simulink model "dynamics_with_control"  (R2023b)
settings: Solver=ode45  StartTime=0.0  StopTime=StopTime  FixedStep=.1  RelTol=1e-5
PreLoadFcn:
  | gravity = true;
  | e_a = 504;
  | e_b = 496;
  | k = 10;
  | b = 10;
  | ktr = 10;
  | btr = 10;
  | ks = 0.1;
  | bs = 10;
  | d0 = 125;
  | l0 = 615.3882;
  | p0 = 100;
  | ls0 = 707.1068;
  | w = -0.007;
  | kp_M = 0.1;
  | ki_M = 0.0023;
  | mu = 398600000000000;
  | mp = 1500;
  | mp_inv = 0.00066667;
  | mtr = 1.6667;
  | mtr_inv = 0.6;
  | NRao0 = [499.999999999579;-4.21217266566732e-10;6878000];
  | NRbo0 = [-500.000000000421;-4.21094801886817e-10;6878000];
  | NRfo0 = [-4.21186650396753e-10;-4.21186650396753e-10;6878500];
  | NRgo0 = [-4.21125418056796e-10;-4.21125418056796e-10;6877500];
  | NRdo0 = [-4.21171342311764e-10;-125.000000000421;6878000];
  | NReo0 = [-4.21140726141785e-10;124.999999999579;6878000];
  | NVao0 = [7612.67977015526;-9.32070078155593e-13;-3.49999999999953];
  | NVbo0 = [7612.67977015526;-9.32498704535295e-13;3.50000000000047];
  | NVfo0 = [7616.17977015526;-9.32713017725146e-13;4.66356508862573e-13];
  | NVgo0 = [7609.17977015526;-9.31855764965743e-13;4.65927882482871e-13];
  | NVdo0 = [7612.67977015526;-9.32284391345444e-13;4.66142195672722e-13];
  | NVeo0 = [7612.67977015526;-9.32284391345444e-13;4.66142195672722e-13];
PostLoadFcn:
  | StopTime = 3000;
values from neighbouring files (symbols this model uses):
  truss_length = 250    [main.m]
libraries: matrix_library x16, vrlib x14
(part 1 of 2)
settings Model: Creator=cyrus  LastModifiedBy=cyrus

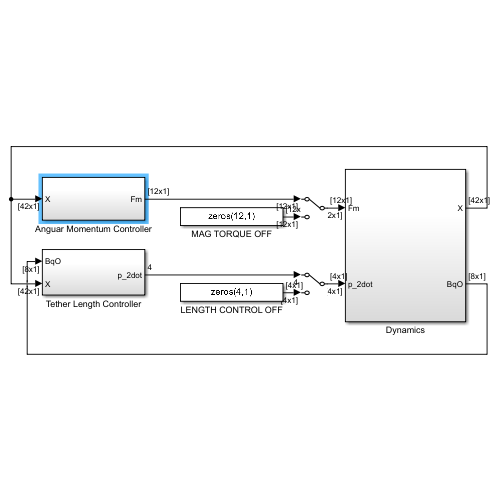
[thumbnail: Simulink's stored preview of the top-level diagram]
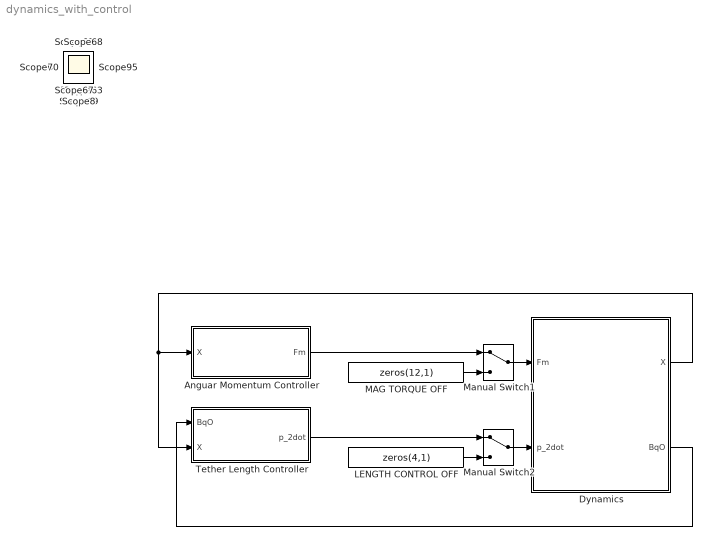
== system dynamics_with_control ==
  Anguar Momentum Controller : Subsystem
  Dynamics : Subsystem
  LENGTH CONTROL OFF : Constant  Value=zeros(4,1)  VectorParams1D=off
  MAG TORQUE OFF : Constant  Value=zeros(12,1)  VectorParams1D=off
  Manual Switch1 : ManualSwitch
  Manual Switch2 : ManualSwitch
  Tether Length Controller : Subsystem
  Scope{,1..36,38,40..70} (69 alike) : Scope
  wires:
  Dynamics/1(X) -> Anguar Momentum Controller/1(X), Tether Length Controller/2(X)
  Manual Switch1/1 -> Dynamics/1(Fm)
  Anguar Momentum Controller/1(Fm) -> Manual Switch1/1
  MAG TORQUE OFF/1 -> Manual Switch1/2
  Manual Switch2/1 -> Dynamics/2(p_2dot)
  LENGTH CONTROL OFF/1 -> Manual Switch2/2
  Tether Length Controller/1(p_2dot) -> Manual Switch2/1
  Dynamics/2(BqO) -> Tether Length Controller/1(BqO)

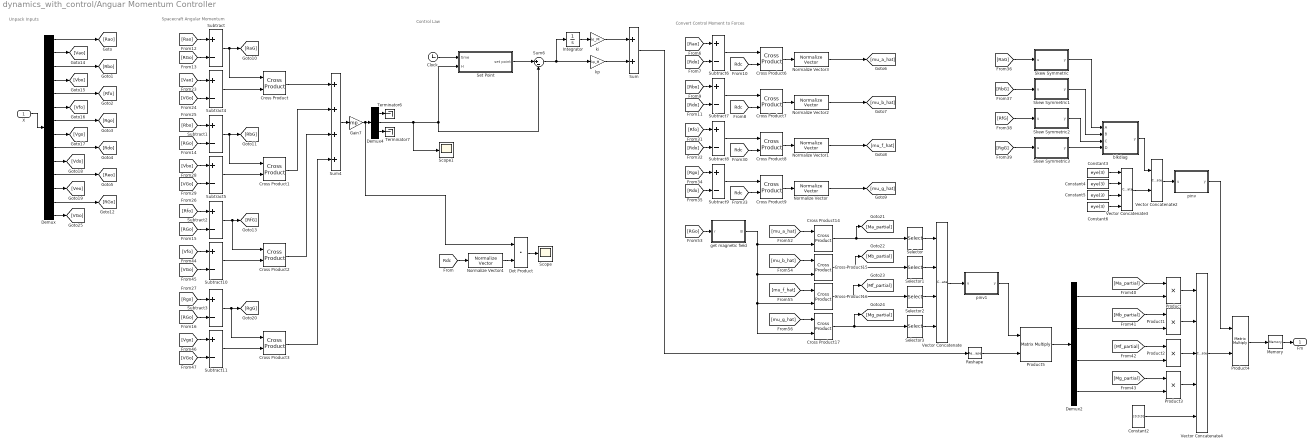
== system dynamics_with_control/Anguar Momentum Controller ==
  note: Convert Control Moment to Forces
  note: Control Law
  note: Spacecraft Angular Momentum
  note: Unpack Inputs
  X : Inport
  Clock : Clock
  Constant2 : Constant  Value=[0;0;0]  VectorParams1D=off
  Constant{3..6} (4 alike) : Constant  Value=eye(3)  VectorParams1D=off
  Cross Product{,1..3,6..9,14..17} (12 alike) : matrix_library/Cross Product
  Demux : Demux  Outputs=14
  Demux2 : Demux
  Demux4 : Demux  Outputs=3
  Dot Product : DotProduct  OutDataTypeStr=Inherit: Inherit via internal rule
  Gain7 : Gain  Gain=mp
  Integrator : Integrator
  Memory : Memory
  Normalize Vector{,1..4} (5 alike) : vrlib/Utilities/Normalize Vector  maxzero=0
  Product{,1..3} (4 alike) : Product
  Product4 : Product  Multiplication=Matrix(*)
  Product5 : Product  Multiplication=Matrix(*)
  Reshape : Reshape  OutputDimensionality=Customize
  Scope : Scope
  Scope1 : Scope
  Selector{,1..3} (4 alike) : Selector  InputPortWidth=3  IndexOptions=Index vector (dialog)  Indices=2  OutputSizes=1
  Set Point : Subsystem
  Skew Symmetric : MATLAB Function  TreatAsAtomicUnit=on
  Skew Symmetric1 : MATLAB Function  TreatAsAtomicUnit=on
  Skew Symmetric2 : MATLAB Function  TreatAsAtomicUnit=on
  Skew Symmetric3 : MATLAB Function  TreatAsAtomicUnit=on
  Subtract{,1..11} (12 alike) : Sum  Inputs=+-
  Sum : Sum
  Sum4 : Sum  Inputs=++++
  Sum6 : Sum  Inputs=|+-
  Terminator6 : Terminator
  Terminator7 : Terminator
  Vector Concatenate : Concatenate  NumInputs=4  Mode=Multidimensional array  ConcatenateDimension=2
  Vector Concatenate2 : Concatenate  Mode=Multidimensional array
  Vector Concatenate3 : Concatenate  NumInputs=4  Mode=Multidimensional array  ConcatenateDimension=2
  Vector Concatenate4 : Concatenate  NumInputs=5
  blkdiag : MATLAB Function  TreatAsAtomicUnit=on
  get magnetic field : MATLAB Function  TreatAsAtomicUnit=on
  ki : Gain  Gain=ki_M
  kp : Gain  Gain=kp_M
  pinv : MATLAB Function  TreatAsAtomicUnit=on
  pinv1 : MATLAB Function  TreatAsAtomicUnit=on
  Fm : Outport
  wires:
  X/1 -> Demux/1
  Sum6/1 -> Integrator/1, kp/1
  Integrator/1 -> ki/1
  ki/1 -> Sum/1
  [RGo] -> Subtract1/2
  Demux/4 -> [Vbo]
  Demux/9 -> [Rdo]
  Demux/2 -> [Vao]
  Subtract3/1 -> Cross Product3/1, [RgG]
  Demux/8 -> [Vgo]
  Demux/10 -> [Vdo]
  Demux/12 -> [Veo]
  Demux/5 -> [Rfo]
  Subtract/1 -> [RaG], Cross Product/1
  Demux/3 -> [Rbo]
  [RGo] -> Subtract3/2
  Demux/7 -> [Rgo]
  Demux/6 -> [Vfo]
  [Rfo] -> Subtract2/1
  Demux/1 -> [Rao]
  [Rbo] -> Subtract1/1
  [RGo] -> Subtract/2
  [Rao] -> Subtract/1
  Subtract1/1 -> Cross Product1/1, [RbG]
  Subtract2/1 -> Cross Product2/1, [RfG]
  Demux/11 -> [Reo]
  [Rgo] -> Subtract3/1
  [RGo] -> Subtract2/2
  [Rdo] -> Subtract6/2
  [Rao] -> Subtract6/1
  Subtract6/1 -> Cross Product6/1
  [Rdc] -> Cross Product6/2
  Cross Product6/1 -> Normalize Vector3/1
  [Rdo] -> Subtract7/2
  [Rbo] -> Subtract7/1
  [Rdc] -> Cross Product7/2
  Subtract7/1 -> Cross Product7/1
  [Rdo] -> Subtract8/2
  [Rfo] -> Subtract8/1
  [Rdc] -> Cross Product8/2
  Cross Product8/1 -> Normalize Vector1/1
  Subtract8/1 -> Cross Product8/1
  [Rdo] -> Subtract9/2
  [Rgo] -> Subtract9/1
  [Rdc] -> Cross Product9/2
  Subtract9/1 -> Cross Product9/1
  Normalize Vector1/1 -> [mu_f_hat]
  Normalize Vector3/1 -> [mu_a_hat]
  Sum4/1 -> Gain7/1
  Demux4/1 -> Terminator6/1
  Demux4/3 -> Terminator7/1
  Sum/1 -> Reshape/1
  [mu_a_hat] -> Cross Product14/1
  [RGo] -> get magnetic field/1(r)
  get magnetic field/1(B) -> Cross Product14/2, Cross Product17/2, Cross Product16/2, Cross Product15/2
  Cross Product14/1 -> [Ma_partial], Selector/1
  Cross Product15/1 -> [Mb_partial], Selector1/1
  [mu_b_hat] -> Cross Product15/1
  [mu_f_hat] -> Cross Product16/1
  [mu_g_hat] -> Cross Product17/1
  Cross Product16/1 -> [Mf_partial], Selector2/1
  Cross Product17/1 -> [Mg_partial], Selector3/1
  Constant2/1 -> Vector Concatenate4/5
  Memory/1 -> Fm/1
  Skew Symmetric/1(y) -> blkdiag/1(A)
  Skew Symmetric1/1(y) -> blkdiag/2(B)
  Skew Symmetric2/1(y) -> blkdiag/3(C)
  Skew Symmetric3/1(y) -> blkdiag/4(D)
  blkdiag/1(y) -> Vector Concatenate2/1
  Vector Concatenate3/1 -> Vector Concatenate2/2
  Constant3/1 -> Vector Concatenate3/1
  Constant4/1 -> Vector Concatenate3/2
  Constant5/1 -> Vector Concatenate3/3
  Constant6/1 -> Vector Concatenate3/4
  [Mb_partial] -> Product1/1
  [Mf_partial] -> Product2/1
  [Mg_partial] -> Product3/1
  Product/1 -> Vector Concatenate4/1
  Product1/1 -> Vector Concatenate4/2
  Product2/1 -> Vector Concatenate4/3
  Product3/1 -> Vector Concatenate4/4
  Vector Concatenate2/1 -> pinv/1(u)
  pinv/1(y) -> Product4/1
  Product4/1 -> Memory/1
  Normalize Vector2/1 -> [mu_b_hat]
  Normalize Vector/1 -> [mu_g_hat]
  Cross Product7/1 -> Normalize Vector2/1
  Cross Product9/1 -> Normalize Vector/1
  [Ma_partial] -> Product/1
  kp/1 -> Sum/2
  Demux4/2 -> Scope1/1, Sum6/2, Set Point/2(H)
  Selector/1 -> Vector Concatenate/1
  Selector3/1 -> Vector Concatenate/4
  Selector2/1 -> Vector Concatenate/3
  Selector1/1 -> Vector Concatenate/2
  Vector Concatenate/1 -> pinv1/1(u)
  pinv1/1(y) -> Product5/1
  Reshape/1 -> Product5/2
  Product5/1 -> Demux2/1
  Demux2/3 -> Product2/2
  Demux2/4 -> Product3/2
  Demux2/2 -> Product1/2
  Demux2/1 -> Product/2
  Vector Concatenate4/1 -> Product4/2
  [RaG] -> Skew Symmetric/1(u)
  [RbG] -> Skew Symmetric1/1(u)
  [RfG] -> Skew Symmetric2/1(u)
  [RgG] -> Skew Symmetric3/1(u)
  Subtract4/1 -> Cross Product/2
  [VGo] -> Subtract4/2
  [Vao] -> Subtract4/1
  [VGo] -> Subtract5/2
  Subtract5/1 -> Cross Product1/2
  [Vbo] -> Subtract5/1
  [Vfo] -> Subtract10/1
  [VGo] -> Subtract10/2
  Subtract10/1 -> Cross Product2/2
  [Vgo] -> Subtract11/1
  [VGo] -> Subtract11/2
  Subtract11/1 -> Cross Product3/2
  Cross Product1/1 -> Sum4/2
  Cross Product2/1 -> Sum4/3
  Cross Product3/1 -> Sum4/4
  Clock/1 -> Set Point/1(time)
  Set Point/1(set point) -> Sum6/1
  Cross Product/1 -> Sum4/1
  Demux/13 -> [RGo]
  Demux/14 -> [VGo]
  Gain7/1 -> Dot Product/1, Demux4/1
  [Rdc] -> Normalize Vector4/1
  Dot Product/1 -> Scope/1
  Normalize Vector4/1 -> Dot Product/2

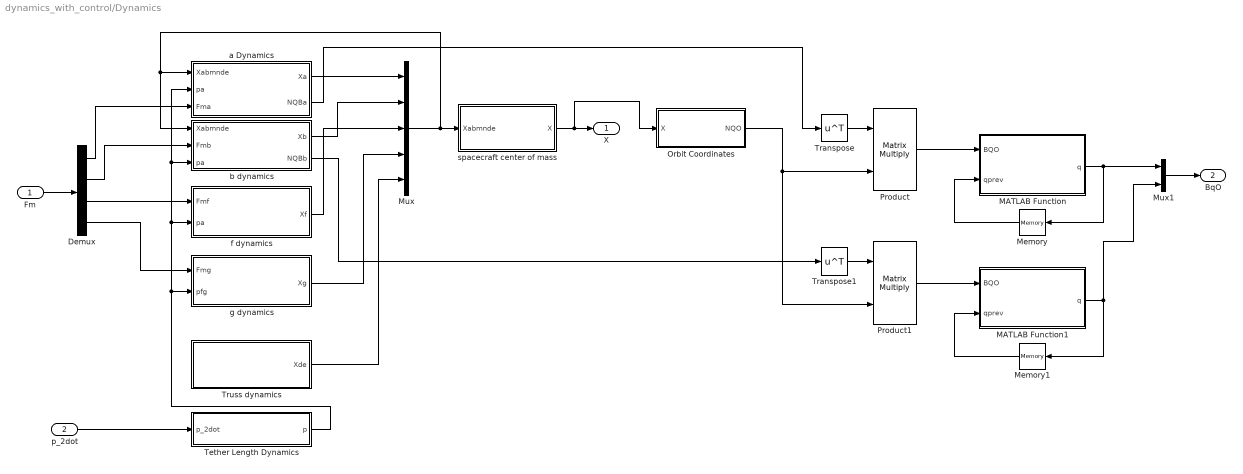
== system dynamics_with_control/Dynamics ==
  Fm : Inport
  p_2dot : Inport  Port=2
  Demux : Demux
  MATLAB Function : MATLAB Function  TreatAsAtomicUnit=on
  MATLAB Function1 : MATLAB Function  TreatAsAtomicUnit=on
  Memory : Memory
  Memory1 : Memory
  Mux : Mux  Inputs=5
  Mux1 : Mux  Inputs=2
  Orbit Coordinates : Subsystem
  Product : Product  Multiplication=Matrix(*)
  Product1 : Product  Multiplication=Matrix(*)
  Tether Length Dynamics : Subsystem
  Transpose : Math  Operator=transpose
  Transpose1 : Math  Operator=transpose
  Truss dynamics : Subsystem
  a Dynamics : Subsystem
  b dynamics : Subsystem
  f dynamics : Subsystem
  g dynamics : Subsystem
  spacecraft center of mass : Subsystem
  X : Outport
  BqO : Outport  Port=2
  wires:
  Mux/1 -> spacecraft center of mass/1(Xabmnde), b dynamics/1(Xabmnde), a Dynamics/1(Xabmnde)
  a Dynamics/1(Xa) -> Mux/1
  b dynamics/1(Xb) -> Mux/2
  f dynamics/1(Xf) -> Mux/3
  g dynamics/1(Xg) -> Mux/4
  Truss dynamics/1(Xde) -> Mux/5
  Demux/1 -> a Dynamics/3(Fma)
  Demux/2 -> b dynamics/2(Fmb)
  Demux/3 -> f dynamics/1(Fmf)
  Demux/4 -> g dynamics/1(Fmg)
  Fm/1 -> Demux/1
  spacecraft center of mass/1(X) -> X/1, Orbit Coordinates/1(X)
  Orbit Coordinates/1(NQO) -> Product/2, Product1/2
  MATLAB Function/1(q) -> Mux1/1, Memory/1
  Memory/1 -> MATLAB Function/2(qprev)
  Product1/1 -> MATLAB Function1/1(BQO)
  Memory1/1 -> MATLAB Function1/2(qprev)
  MATLAB Function1/1(q) -> Mux1/2, Memory1/1
  Mux1/1 -> BqO/1
  Product/1 -> MATLAB Function/1(BQO)
  a Dynamics/2(NQBa) -> Transpose/1
  Transpose/1 -> Product/1
  Transpose1/1 -> Product1/1
  b dynamics/2(NQBb) -> Transpose1/1
  Tether Length Dynamics/1(p) -> a Dynamics/2(pa), b dynamics/3(pa), f dynamics/2(pa), g dynamics/2(pfg)
  p_2dot/1 -> Tether Length Dynamics/1(p_2dot)

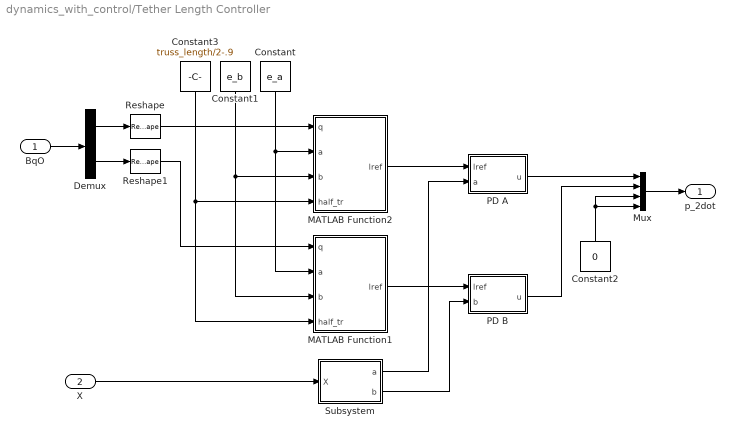
== system dynamics_with_control/Tether Length Controller ==
  BqO : Inport
  X : Inport  Port=2
  Constant : Constant  Value=e_a
  Constant1 : Constant  Value=e_b
  Constant2 : Constant  Value=0
  Constant3 : Constant  Value=truss_length/2-.9
  Demux : Demux  Outputs=2
  MATLAB Function1 : MATLAB Function  TreatAsAtomicUnit=on
  MATLAB Function2 : MATLAB Function  TreatAsAtomicUnit=on
  Mux : Mux
  PD A : Subsystem
  PD B : Subsystem
  Reshape : Reshape  OutputDimensionality=Customize  OutputDimensions=[4,1]
  Reshape1 : Reshape  OutputDimensionality=Customize  OutputDimensions=[4,1]
  Subsystem : Subsystem
  p_2dot : Outport
  wires:
  Mux/1 -> p_2dot/1
  BqO/1 -> Demux/1
  Demux/1 -> Reshape/1
  PD A/1(u) -> Mux/1
  Constant/1 -> MATLAB Function2/2(a), MATLAB Function1/2(a)
  Constant1/1 -> MATLAB Function2/3(b), MATLAB Function1/3(b)
  Demux/2 -> Reshape1/1
  Constant3/1 -> MATLAB Function2/4(half_tr), MATLAB Function1/4(half_tr)
  PD B/1(u) -> Mux/2
  Constant2/1 -> Mux/4, Mux/3
  Reshape/1 -> MATLAB Function2/1(q)
  Reshape1/1 -> MATLAB Function1/1(q)
  X/1 -> Subsystem/1(X)
  MATLAB Function2/1(lref) -> PD A/1(lref)
  MATLAB Function1/1(lref) -> PD B/1(lref)
  Subsystem/1(a) -> PD A/2(a)
  Subsystem/2(b) -> PD B/2(b)

== system dynamics_with_control/Anguar Momentum Controller/Set Point ==
  time : Inport
  H : Inport  Port=2
  Memory1 : Memory
  Switch : Switch  Criteria=u2 > Threshold  SaturateOnIntegerOverflow=off  InputSameDT=off
  set point : Outport
  wires:
  Memory1/1 -> Switch/1
  time/1 -> Switch/2
  H/1 -> Switch/3
  Switch/1 -> set point/1, Memory1/1

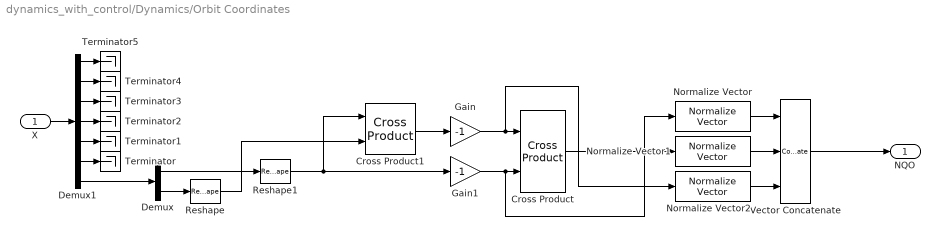
== system dynamics_with_control/Dynamics/Orbit Coordinates ==
  X : Inport
  Cross Product : matrix_library/Cross Product
  Cross Product1 : matrix_library/Cross Product
  Demux : Demux  Outputs=2
  Demux1 : Demux  Outputs=7
  Gain : Gain  Gain=-1
  Gain1 : Gain  Gain=-1
  Normalize Vector : vrlib/Utilities/Normalize Vector  maxzero=0
  Normalize Vector1 : vrlib/Utilities/Normalize Vector  maxzero=0
  Normalize Vector2 : vrlib/Utilities/Normalize Vector  maxzero=0
  Reshape : Reshape  OutputDimensionality=Column vector (2-D)
  Reshape1 : Reshape  OutputDimensionality=Column vector (2-D)
  Terminator{,1..5} (6 alike) : Terminator
  Vector Concatenate : Concatenate  NumInputs=3  Mode=Multidimensional array  ConcatenateDimension=2
  NQO : Outport
  wires:
  Normalize Vector/1 -> Vector Concatenate/1
  Normalize Vector1/1 -> Vector Concatenate/2
  Normalize Vector2/1 -> Vector Concatenate/3
  Vector Concatenate/1 -> NQO/1
  Demux/1 -> Reshape1/1
  Demux/2 -> Reshape/1
  Cross Product1/1 -> Gain/1
  Gain/1 -> Normalize Vector2/1, Cross Product/1
  Gain1/1 -> Normalize Vector/1, Cross Product/2
  Reshape1/1 -> Gain1/1, Cross Product1/1
  Reshape/1 -> Cross Product1/2
  Cross Product/1 -> Normalize Vector1/1
  X/1 -> Demux1/1
  Demux1/7 -> Demux/1
  Demux1/6 -> Terminator/1
  Demux1/5 -> Terminator1/1
  Demux1/4 -> Terminator2/1
  Demux1/3 -> Terminator3/1
  Demux1/2 -> Terminator4/1
  Demux1/1 -> Terminator5/1

== system dynamics_with_control/Dynamics/Tether Length Dynamics ==
  p_2dot : Inport
  Demux : Demux
  Integrator{,2,4,6} (4 alike) : Integrator
  Integrator{1,3,5,7} (4 alike) : Integrator  InitialCondition=p0
  Mux{,1..3} (4 alike) : Mux  Inputs=2
  Mux4 : Mux
  p : Outport
  wires:
  Integrator/1 -> Mux/2, Integrator1/1
  p_2dot/1 -> Demux/1
  Integrator2/1 -> Mux1/2, Integrator3/1
  Integrator4/1 -> Mux2/2, Integrator5/1
  Integrator6/1 -> Mux3/2, Integrator7/1
  Integrator1/1 -> Mux/1
  Integrator7/1 -> Mux3/1
  Integrator5/1 -> Mux2/1
  Integrator3/1 -> Mux1/1
  Mux/1 -> Mux4/1
  Mux1/1 -> Mux4/2
  Mux2/1 -> Mux4/3
  Mux3/1 -> Mux4/4
  Mux4/1 -> p/1
  Demux/1 -> Integrator/1
  Demux/2 -> Integrator2/1
  Demux/3 -> Integrator4/1
  Demux/4 -> Integrator6/1

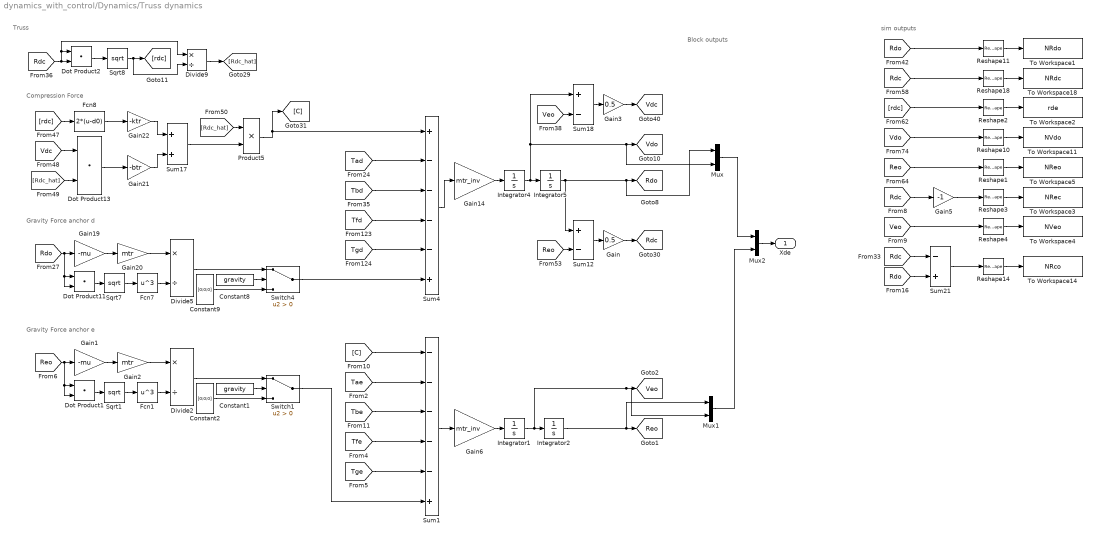
== system dynamics_with_control/Dynamics/Truss dynamics ==
  note: Block outputs
  note: Truss
  note: Gravity Force anchor d
  note: Compression Force
  note: sim outputs
  note: Gravity Force anchor e
  Constant1 : Constant  Value=gravity
  Constant2 : Constant  Value=[0;0;0]  VectorParams1D=off
  Constant8 : Constant  Value=gravity
  Constant9 : Constant  Value=[0;0;0]  VectorParams1D=off
  Divide2 : Product  Inputs=*/
  Divide5 : Product  Inputs=*/
  Divide9 : Product  Inputs=*/
  Dot Product{1..2,11,13} (4 alike) : DotProduct  OutDataTypeStr=Inherit: Inherit via internal rule
  Fcn1 : Fcn  Expr=u^3
  Fcn7 : Fcn  Expr=u^3
  Fcn8 : Fcn  Expr=2*(u-d0)
  Gain : Gain  Gain=0.5
  Gain1 : Gain  Gain=-mu
  Gain14 : Gain  Gain=mtr_inv
  Gain19 : Gain  Gain=-mu
  Gain2 : Gain  Gain=mtr
  Gain20 : Gain  Gain=mtr
  Gain21 : Gain  Gain=-btr
  Gain22 : Gain  Gain=-ktr
  Gain3 : Gain  Gain=0.5
  Gain5 : Gain  Gain=-1
  Gain6 : Gain  Gain=mtr_inv
  Integrator1 : Integrator  InitialCondition=NVeo0
  Integrator2 : Integrator  InitialCondition=NReo0
  Integrator4 : Integrator  InitialCondition=NVdo0
  Integrator5 : Integrator  InitialCondition=NRdo0
  Mux : Mux  Inputs=2
  Mux1 : Mux  Inputs=2
  Mux2 : Mux  Inputs=2
  Product5 : Product
  Reshape{1..4,10..11,14,18} (8 alike) : Reshape
  Sqrt1 : Sqrt
  Sqrt7 : Sqrt
  Sqrt8 : Sqrt
  Sum1 : Sum  Inputs=-----+
  Sum12 : Sum  Inputs=+-
  Sum17 : Sum
  Sum18 : Sum  Inputs=+-
  Sum21 : Sum  Inputs=-+
  Sum4 : Sum  Inputs=+----+
  Switch1 : Switch  Criteria=u2 > Threshold  SaturateOnIntegerOverflow=off  InputSameDT=off
  Switch4 : Switch  Criteria=u2 > Threshold  SaturateOnIntegerOverflow=off  InputSameDT=off
  To Workspace1 : ToWorkspace  VariableName=NRdo  SampleTime=-1
      settings: Save2DSignal=2-D array (concatenate along first dimension)
  To Workspace11 : ToWorkspace  VariableName=NVdo  SampleTime=-1
      settings: Save2DSignal=2-D array (concatenate along first dimension)
  To Workspace14 : ToWorkspace  VariableName=NRco  SampleTime=-1
      settings: Save2DSignal=2-D array (concatenate along first dimension)
  To Workspace18 : ToWorkspace  VariableName=NRdc  SampleTime=-1
      settings: Save2DSignal=2-D array (concatenate along first dimension)
  To Workspace2 : ToWorkspace  VariableName=rde  SampleTime=-1
      settings: Save2DSignal=2-D array (concatenate along first dimension)
  To Workspace3 : ToWorkspace  VariableName=NRec  SampleTime=-1
      settings: Save2DSignal=2-D array (concatenate along first dimension)
  To Workspace4 : ToWorkspace  VariableName=NVeo  SampleTime=-1
      settings: Save2DSignal=2-D array (concatenate along first dimension)
  To Workspace5 : ToWorkspace  VariableName=NReo  SampleTime=-1
      settings: Save2DSignal=2-D array (concatenate along first dimension)
  Xde : Outport
  tag scope: Rdc=global, Rdo=global, Reo=global, Vdc=global, Vdo=global, Veo=global
  wires:
  [Veo] -> Sum18/2
  [Tad] -> Sum4/2
  [Tbd] -> Sum4/3
  Constant8/1 -> Switch4/2
  Sum4/1 -> Gain14/1
  Gain14/1 -> Integrator4/1
  Constant9/1 -> Switch4/3
  Product5/1 -> [C], Sum4/1
  Gain/1 -> [Rdc]
  [Tgd] -> Sum4/5
  Fcn8/1 -> Gain22/1
  Integrator5/1 -> Mux/1, [Rdo], Sum12/1
  [Vdc] -> Dot Product13/1
  Gain22/1 -> Sum17/1
  Fcn7/1 -> Divide5/2
  [Rdc_hat] -> Dot Product13/2
  [Rdc_hat] -> Product5/1
  Gain20/1 -> Divide5/1
  [Reo] -> Sum12/2
  Sum12/1 -> Gain/1
  Integrator4/1 -> Integrator5/1, Sum18/1, Mux/2, [Vdo]
  Divide5/1 -> Switch4/1
  [Tfd] -> Sum4/4
  Sqrt8/1 -> Divide9/2, [rdc]
  Sqrt7/1 -> Fcn7/1
  [Rdc] -> Divide9/1, Dot Product2/1, Dot Product2/2
  Switch4/1 -> Sum4/6
  [Rdo] -> Dot Product11/2, Dot Product11/1, Gain19/1
  Dot Product11/1 -> Sqrt7/1
  Gain19/1 -> Gain20/1
  Sum17/1 -> Product5/2
  Dot Product2/1 -> Sqrt8/1
  Dot Product13/1 -> Gain21/1
  Divide9/1 -> [Rdc_hat]
  Gain21/1 -> Sum17/2
  [rdc] -> Fcn8/1
  [Vdo] -> Reshape10/1
  [Rdo] -> Reshape11/1
  [rdc] -> Reshape2/1
  Reshape10/1 -> To Workspace11/1
  Reshape18/1 -> To Workspace18/1
  Reshape11/1 -> To Workspace1/1
  [Rdc] -> Reshape18/1
  Reshape2/1 -> To Workspace2/1
  Reshape1/1 -> To Workspace5/1
  [Reo] -> Reshape1/1
  [Rdc] -> Sum21/1
  [Rdo] -> Sum21/2
  Sum21/1 -> Reshape14/1
  Reshape14/1 -> To Workspace14/1
  Sum18/1 -> Gain3/1
  Gain3/1 -> [Vdc]
  Reshape3/1 -> To Workspace3/1
  Gain5/1 -> Reshape3/1
  [Rdc] -> Gain5/1
  Reshape4/1 -> To Workspace4/1
  [Veo] -> Reshape4/1
  Dot Product1/1 -> Sqrt1/1
  Switch1/1 -> Sum1/6
  Integrator2/1 -> Mux1/1, [Reo]
  Integrator1/1 -> Mux1/2, [Veo], Integrator2/1
  Gain6/1 -> Integrator1/1
  [Tge] -> Sum1/5
  Constant1/1 -> Switch1/2
  Gain2/1 -> Divide2/1
  [Tae] -> Sum1/2
  Sum1/1 -> Gain6/1
  [Tbe] -> Sum1/3
  [C] -> Sum1/1
  Constant2/1 -> Switch1/3
  Gain1/1 -> Gain2/1
  Sqrt1/1 -> Fcn1/1
  [Tfe] -> Sum1/4
  [Reo] -> Dot Product1/2, Dot Product1/1, Gain1/1
  Fcn1/1 -> Divide2/2
  Divide2/1 -> Switch1/1
  Mux/1 -> Mux2/1
  Mux1/1 -> Mux2/2
  Mux2/1 -> Xde/1

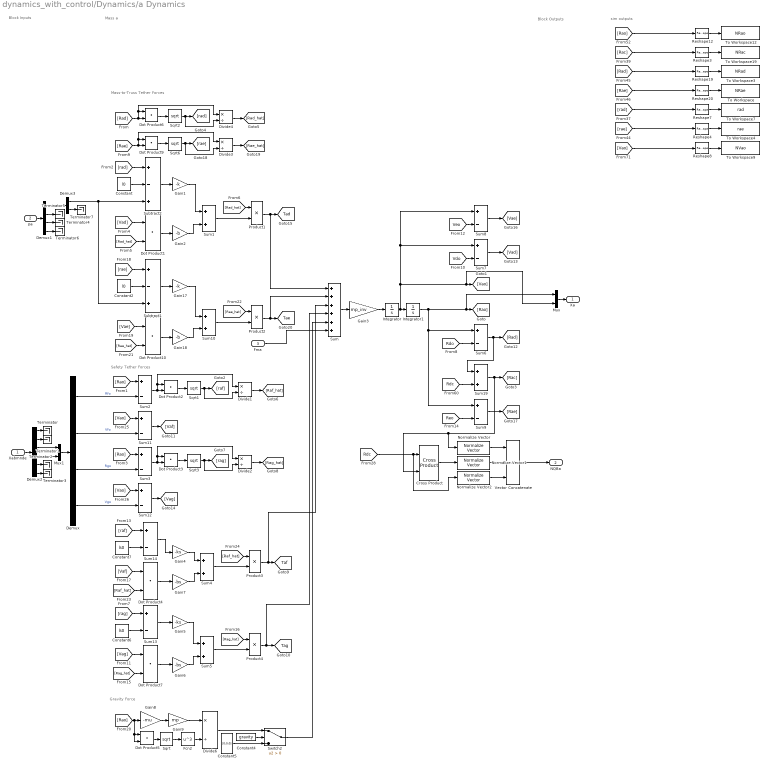
== system dynamics_with_control/Dynamics/a Dynamics ==
  note: Block Inputs
  note: Block Outputs
  note: Mass-to-Truss Tether Forces
  note: Mass a
  note: Gravity Force
  note: sim outputs
  note: Safety Tether Forces
  Xabmnde : Inport
  pa : Inport  Port=2
  Fma : Inport  Port=3
  Constant : Constant  Value=l0
  Constant2 : Constant  Value=l0
  Constant4 : Constant  Value=gravity
  Constant5 : Constant  Value=[0;0;0]  VectorParams1D=off
  Constant6 : Constant  Value=ls0
  Constant7 : Constant  Value=ls0
  Cross Product : matrix_library/Cross Product
  Demux : Demux
  Demux1 : Demux
  Demux2 : Demux  Outputs=6
  Demux3 : Demux  Outputs=2
  Divide{1..4,6} (5 alike) : Product  Inputs=*/
  Dot Product{1..7,9..10} (9 alike) : DotProduct  OutDataTypeStr=Inherit: Inherit via internal rule
  Fcn2 : Fcn  Expr=u^3
  Gain1 : Gain  Gain=-k
  Gain17 : Gain  Gain=-k
  Gain18 : Gain  Gain=-b
  Gain2 : Gain  Gain=-b
  Gain3 : Gain  Gain=mp_inv
  Gain4 : Gain  Gain=-ks
  Gain5 : Gain  Gain=-ks
  Gain6 : Gain  Gain=-bs
  Gain7 : Gain  Gain=-bs
  Gain8 : Gain  Gain=-mu
  Gain9 : Gain  Gain=mp
  Integrator : Integrator  InitialCondition=NVao0
  Integrator1 : Integrator  InitialCondition=NRao0
  Mux : Mux  Inputs=2
  Mux1 : Mux  Inputs=2
  Normalize Vector : vrlib/Utilities/Normalize Vector  maxzero=0
  Normalize Vector1 : vrlib/Utilities/Normalize Vector  maxzero=0
  Normalize Vector2 : vrlib/Utilities/Normalize Vector  maxzero=0
  Product{1..4} (4 alike) : Product
  Reshape{3..4,7..8,12,19..20} (7 alike) : Reshape
  Sqrt{,1..3,6} (5 alike) : Sqrt
  Subtract1 : Sum  Inputs=+-+
  Subtract2 : Sum  Inputs=+-+
  Sum : Sum  Inputs=++++++
  Sum{1,4..5,10,19} (5 alike) : Sum
  Sum{2..3,6..9,11..14} (10 alike) : Sum  Inputs=+-
  Switch2 : Switch  Criteria=u2 > Threshold  SaturateOnIntegerOverflow=off  InputSameDT=off
  Terminator{,1..7} (8 alike) : Terminator
  To Workspace : ToWorkspace  VariableName=NRae  SampleTime=-1
  To Workspace12 : ToWorkspace  VariableName=NRao  SampleTime=-1
      settings: Save2DSignal=2-D array (concatenate along first dimension)
  To Workspace19 : ToWorkspace  VariableName=NRac  SampleTime=-1
      settings: Save2DSignal=2-D array (concatenate along first dimension)
  To Workspace3 : ToWorkspace  VariableName=NRad  SampleTime=-1
  To Workspace4 : ToWorkspace  VariableName=rae  SampleTime=-1
      settings: Save2DSignal=2-D array (concatenate along first dimension)
  To Workspace7 : ToWorkspace  VariableName=rad  SampleTime=-1
      settings: Save2DSignal=2-D array (concatenate along first dimension)
  To Workspace9 : ToWorkspace  VariableName=NVao  SampleTime=-1
      settings: Save2DSignal=2-D array (concatenate along first dimension)
  Vector Concatenate : Concatenate  NumInputs=3  Mode=Multidimensional array  ConcatenateDimension=2
  Xa : Outport
  NQBa : Outport  Port=2
  tag scope: Tad=global, Tae=global, Taf=global, Tag=global
  wires:
  Sum19/1 -> Normalize Vector/1, Cross Product/2, [Rac]
  [Rdo] -> Sum6/2
  Dot Product6/1 -> Sqrt2/1
  Gain17/1 -> Sum10/1
  [Veo] -> Sum8/2
  Dot Product10/1 -> Gain18/1
  Dot Product5/1 -> Sqrt/1
  Gain18/1 -> Sum10/2
  Sum1/1 -> Product1/2
  Sqrt/1 -> Fcn2/1
  [Rad_hat] -> Product1/1
  Sum9/1 -> [Rae]
  Constant5/1 -> Switch2/3
  Gain2/1 -> Sum1/2
  Sqrt2/1 -> Divide4/2, [rad]
  Sum8/1 -> [Vae]
  [Rae_hat] -> Dot Product10/2
  Sum/1 -> Gain3/1
  Integrator1/1 -> Mux/1, [Rao], Sum9/1, Sum6/1
  Fcn2/1 -> Divide6/2
  [rad] -> Subtract2/1
  [Rae_hat] -> Product2/1
  Gain3/1 -> Integrator/1
  Gain9/1 -> Divide6/1
  [Rad_hat] -> Dot Product1/2
  Divide4/1 -> [Rad_hat]
  [Rao] -> Dot Product5/2, Dot Product5/1, Gain8/1
  Product2/1 -> Sum/2, [Tae]
  [Rad] -> Divide4/1, Dot Product6/1, Dot Product6/2
  Subtract2/1 -> Gain1/1
  Constant4/1 -> Switch2/2
  Gain1/1 -> Sum1/1
  [Vad] -> Dot Product1/1
  Sum10/1 -> Product2/2
  [Reo] -> Sum9/2
  Dot Product1/1 -> Gain2/1
  Switch2/1 -> Sum/5
  Gain8/1 -> Gain9/1
  Sum7/1 -> [Vad]
  [Rae] -> Divide3/1, Dot Product9/1, Dot Product9/2
  [Rdc] -> Sum19/2
  Sqrt6/1 -> Divide3/2, [rae]
  Divide6/1 -> Switch2/1
  [Vdo] -> Sum7/2
  Product1/1 -> Sum/1, [Tad]
  Dot Product9/1 -> Sqrt6/1
  Integrator/1 -> Integrator1/1, Mux/2, [Vao], Sum7/1, Sum8/1
  Divide3/1 -> [Rae_hat]
  Sum6/1 -> Sum19/1, [Rad]
  [Vae] -> Dot Product10/1
  Reshape4/1 -> To Workspace4/1
  Reshape19/1 -> To Workspace3/1
  Reshape8/1 -> To Workspace9/1
  Reshape12/1 -> To Workspace12/1
  [Rad] -> Reshape19/1
  Reshape20/1 -> To Workspace/1
  [Rae] -> Reshape20/1
  [rad] -> Reshape7/1
  Reshape7/1 -> To Workspace7/1
  [Vao] -> Reshape8/1
  [Rao] -> Reshape12/1
  [rae] -> Reshape4/1
  [Rac] -> Reshape3/1
  Reshape3/1 -> To Workspace19/1
  [Rao] -> Sum2/1
  Demux/1 -> Sum2/2  "Rfo"
  Dot Product2/1 -> Sqrt1/1
  Sqrt1/1 -> Divide1/2, [raf]
  Divide1/1 -> [Raf_hat]
  Sum2/1 -> Divide1/1, Dot Product2/1, Dot Product2/2
  Demux/2 -> Sum11/2  "Vfo"
  Dot Product7/1 -> Gain6/1
  [Rag_hat] -> Product4/1
  Gain4/1 -> Sum4/1
  Product4/1 -> [Tag], Sum/4
  [Rag_hat] -> Dot Product7/2
  [Raf_hat] -> Product3/1
  Gain7/1 -> Sum4/2
  Sum5/1 -> Product4/2
  [Raf_hat] -> Dot Product4/2
  Gain6/1 -> Sum5/2
  [rag] -> Sum13/1
  Dot Product4/1 -> Gain7/1
  Gain5/1 -> Sum5/1
  [Vaf] -> Dot Product4/1
  Sum13/1 -> Gain5/1
  [Vag] -> Dot Product7/1
  Product3/1 -> Sum/3, [Taf]
  Sum4/1 -> Product3/2
  Demux/3 -> Sum3/2  "Rgo"
  [Vao] -> Sum11/1
  Sum11/1 -> [Vaf]
  [Vao] -> Sum12/1
  Sum12/1 -> [Vag]
  Demux/4 -> Sum12/2  "Vgo"
  Dot Product3/1 -> Sqrt3/1
  Divide2/1 -> [Rag_hat]
  Sqrt3/1 -> Divide2/2, [rag]
  [Rao] -> Sum3/1
  Sum3/1 -> Divide2/1, Dot Product3/1, Dot Product3/2
  Mux/1 -> Xa/1
  Xabmnde/1 -> Demux2/1
  Mux1/1 -> Demux/1
  Demux2/3 -> Mux1/1
  Demux2/4 -> Mux1/2
  Demux2/1 -> Terminator/1
  Demux2/2 -> Terminator1/1
  Demux2/5 -> Terminator2/1
  Demux2/6 -> Terminator3/1
  Constant/1 -> Subtract2/2
  [rae] -> Subtract1/1
  Constant2/1 -> Subtract1/2
  Subtract1/1 -> Gain17/1
  Constant6/1 -> Sum13/2
  [raf] -> Sum14/1
  Constant7/1 -> Sum14/2
  Sum14/1 -> Gain4/1
  Fma/1 -> Sum/6
  Demux1/4 -> Terminator6/1
  Demux1/2 -> Terminator5/1
  Demux1/3 -> Terminator4/1
  pa/1 -> Demux1/1
  Cross Product/1 -> Normalize Vector1/1
  [Rdc] -> Normalize Vector2/1, Cross Product/1
  Normalize Vector/1 -> Vector Concatenate/1
  Normalize Vector1/1 -> Vector Concatenate/2
  Normalize Vector2/1 -> Vector Concatenate/3
  Vector Concatenate/1 -> NQBa/1
  Demux1/1 -> Demux3/1
  Demux3/1 -> Subtract2/3, Subtract1/3
  Demux3/2 -> Terminator7/1

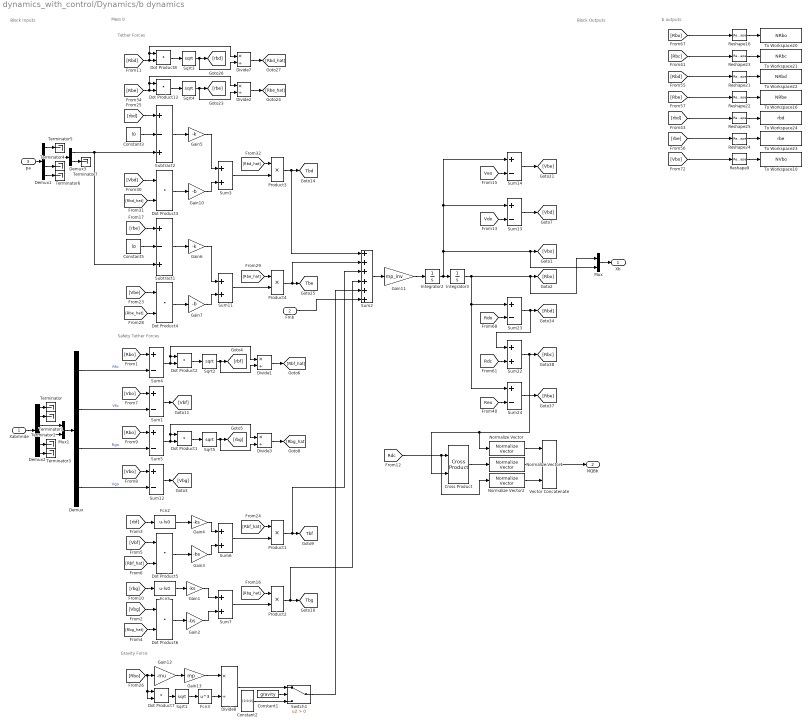
== system dynamics_with_control/Dynamics/b dynamics ==
  note: Gravity Force
  note: Tether Forces
  note: Mass b
  note: b outputs
  note: Safety Tether Forces
  note: Block Inputs
  note: Block Outputs
  Xabmnde : Inport
  Fmb : Inport  Port=2
  pa : Inport  Port=3
  Constant1 : Constant  Value=gravity
  Constant2 : Constant  Value=[0;0;0]  VectorParams1D=off
  Constant3 : Constant  Value=l0
  Constant5 : Constant  Value=l0
  Cross Product : matrix_library/Cross Product
  Demux : Demux
  Demux1 : Demux
  Demux2 : Demux  Outputs=6
  Demux3 : Demux  Outputs=2
  Divide{1..3,7..8} (5 alike) : Product  Inputs=*/
  Dot Product{1..8,12} (9 alike) : DotProduct  OutDataTypeStr=Inherit: Inherit via internal rule
  Fcn2 : Fcn  Expr=u-ls0
  Fcn3 : Fcn  Expr=u^3
  Fcn5 : Fcn  Expr=u-ls0
  Gain1 : Gain  Gain=-ks
  Gain10 : Gain  Gain=-b
  Gain11 : Gain  Gain=mp_inv
  Gain12 : Gain  Gain=-mu
  Gain13 : Gain  Gain=mp
  Gain2 : Gain  Gain=-bs
  Gain3 : Gain  Gain=-bs
  Gain4 : Gain  Gain=-ks
  Gain5 : Gain  Gain=-k
  Gain6 : Gain  Gain=-k
  Gain7 : Gain  Gain=-b
  Integrator2 : Integrator  InitialCondition=NVbo0
  Integrator3 : Integrator  InitialCondition=NRbo0
  Mux : Mux  Inputs=2
  Mux1 : Mux  Inputs=2
  Normalize Vector : vrlib/Utilities/Normalize Vector  maxzero=0
  Normalize Vector1 : vrlib/Utilities/Normalize Vector  maxzero=0
  Normalize Vector2 : vrlib/Utilities/Normalize Vector  maxzero=0
  Product{1..4} (4 alike) : Product
  Reshape{9,16,21..25} (7 alike) : Reshape
  Sqrt{1..5} (5 alike) : Sqrt
  Subtract1 : Sum  Inputs=+-+
  Subtract2 : Sum  Inputs=+-+
  Sum{1,4..5,12..14,23..24} (8 alike) : Sum  Inputs=+-
  Sum{3,6..7,11,22} (5 alike) : Sum
  Sum2 : Sum  Inputs=++++++
  Switch1 : Switch  Criteria=u2 > Threshold  SaturateOnIntegerOverflow=off  InputSameDT=off
  Terminator{,1..7} (8 alike) : Terminator
  To Workspace10 : ToWorkspace  VariableName=NVbo  SampleTime=-1
      settings: Save2DSignal=2-D array (concatenate along first dimension)
  To Workspace16 : ToWorkspace  VariableName=NRbe  SampleTime=-1
  To Workspace20 : ToWorkspace  VariableName=NRbo  SampleTime=-1
      settings: Save2DSignal=2-D array (concatenate along first dimension)
  To Workspace21 : ToWorkspace  VariableName=NRbc  SampleTime=-1
      settings: Save2DSignal=2-D array (concatenate along first dimension)
  To Workspace22 : ToWorkspace  VariableName=NRbd  SampleTime=-1
  To Workspace23 : ToWorkspace  VariableName=rbe  SampleTime=-1
      settings: Save2DSignal=2-D array (concatenate along first dimension)
  To Workspace24 : ToWorkspace  VariableName=rbd  SampleTime=-1
      settings: Save2DSignal=2-D array (concatenate along first dimension)
  Vector Concatenate : Concatenate  NumInputs=3  Mode=Multidimensional array  ConcatenateDimension=2
  Xb : Outport
  NQBb : Outport  Port=2
  tag scope: Tbd=global, Tbe=global, Tbf=global, Tbg=global
  wires:
  Fcn3/1 -> Divide8/2
  Dot Product12/1 -> Sqrt4/1
  [Rbe_hat] -> Dot Product4/2
  Divide8/1 -> Switch1/1
  Gain12/1 -> Gain13/1
  Gain10/1 -> Sum3/2
  Gain13/1 -> Divide8/1
  Product4/1 -> Sum2/2, [Tbe]
  Sum3/1 -> Product3/2
  Dot Product4/1 -> Gain7/1
  Gain11/1 -> Integrator2/1
  [Rbo] -> Dot Product7/2, Dot Product7/1, Gain12/1
  Sum24/1 -> [Rbe]
  [Rbd] -> Divide7/1, Dot Product8/1, Dot Product8/2
  Sqrt1/1 -> Fcn3/1
  Divide2/1 -> [Rbe_hat]
  Sqrt4/1 -> Divide2/2, [rbe]
  [Rbe_hat] -> Product4/1
  Sum13/1 -> [Vbd]
  Dot Product3/1 -> Gain10/1
  Constant2/1 -> Switch1/3
  [Vdo] -> Sum13/2
  [Rbd_hat] -> Product3/1
  Integrator2/1 -> Integrator3/1, Sum14/1, Sum13/1, Mux/2, [Vbo]
  Constant1/1 -> Switch1/2
  Gain5/1 -> Sum3/1
  Integrator3/1 -> Sum24/1, Sum23/1, Mux/1, [Rbo]
  [Vbd] -> Dot Product3/1
  Gain6/1 -> Sum11/1
  [Rdc] -> Sum22/2
  [Vbe] -> Dot Product4/1
  Dot Product7/1 -> Sqrt1/1
  [Veo] -> Sum14/2
  [Rbe] -> Divide2/1, Dot Product12/1, Dot Product12/2
  [Rbd_hat] -> Dot Product3/2
  Sum23/1 -> Sum22/1, [Rbd]
  Dot Product8/1 -> Sqrt3/1
  Switch1/1 -> Sum2/5
  [Reo] -> Sum24/2
  Divide7/1 -> [Rbd_hat]
  Sum2/1 -> Gain11/1
  Gain7/1 -> Sum11/2
  Sum11/1 -> Product4/2
  Sum14/1 -> [Vbe]
  Sqrt3/1 -> Divide7/2, [rbd]
  Product3/1 -> [Tbd], Sum2/1
  [Rdo] -> Sum23/2
  Reshape21/1 -> To Workspace22/1
  Reshape23/1 -> To Workspace21/1
  Reshape9/1 -> To Workspace10/1
  [Rbc] -> Reshape23/1
  Reshape25/1 -> To Workspace24/1
  [Vbo] -> Reshape9/1
  Reshape22/1 -> To Workspace16/1
  [Rbo] -> Reshape16/1
  Reshape24/1 -> To Workspace23/1
  [Rbd] -> Reshape21/1
  [rbd] -> Reshape25/1
  [Rbe] -> Reshape22/1
  Reshape16/1 -> To Workspace20/1
  [rbe] -> Reshape24/1
  Dot Product6/1 -> Gain2/1
  [Rbg_hat] -> Dot Product6/2
  [Rbf_hat] -> Product1/1
  Gain3/1 -> Sum6/2
  Dot Product2/1 -> Sqrt2/1
  Divide1/1 -> [Rbf_hat]
  Sum4/1 -> Divide1/1, Dot Product2/1, Dot Product2/2
  [Vbg] -> Dot Product6/1
  [Vbo] -> Sum12/1
  [rbg] -> Fcn5/1
  [Rbf_hat] -> Dot Product5/2
  [rbf] -> Fcn2/1
  Fcn5/1 -> Gain1/1
  [Rbg_hat] -> Product2/1
  [Vbo] -> Sum1/1
  Sum1/1 -> [Vbf]
  Sum6/1 -> Product1/2
  Gain4/1 -> Sum6/1
  Sum12/1 -> [Vbg]
  Product1/1 -> Sum2/3, [Tbf]
  [Rbo] -> Sum4/1
  Demux/2 -> Sum1/2  "Vfo"
  Demux/4 -> Sum12/2  "Vgo"
  Dot Product5/1 -> Gain3/1
  Sqrt2/1 -> Divide1/2, [rbf]
  Gain1/1 -> Sum7/1
  Sum7/1 -> Product2/2
  Fcn2/1 -> Gain4/1
  [Vbf] -> Dot Product5/1
  Gain2/1 -> Sum7/2
  Product2/1 -> Sum2/4, [Tbg]
  Dot Product1/1 -> Sqrt5/1
  Sqrt5/1 -> Divide3/2, [rbg]
  Sum5/1 -> Divide3/1, Dot Product1/1, Dot Product1/2
  Divide3/1 -> [Rbg_hat]
  Demux/3 -> Sum5/2  "Rgo"
  [Rbo] -> Sum5/1
  Demux/1 -> Sum4/2  "Rfo"
  Mux/1 -> Xb/1
  Demux2/5 -> Terminator2/1
  Demux2/3 -> Mux1/1
  Demux2/4 -> Mux1/2
  Demux2/1 -> Terminator/1
  Demux2/6 -> Terminator3/1
  Demux2/2 -> Terminator1/1
  Mux1/1 -> Demux/1
  Xabmnde/1 -> Demux2/1
  [rbd] -> Subtract2/1
  Subtract2/1 -> Gain5/1
  Constant3/1 -> Subtract2/2
  [rbe] -> Subtract1/1
  Constant5/1 -> Subtract1/2
  Subtract1/1 -> Gain6/1
  Fmb/1 -> Sum2/6
  Demux1/2 -> Demux3/1
  Demux1/3 -> Terminator4/1
  pa/1 -> Demux1/1
  Demux1/4 -> Terminator6/1
  Sum22/1 -> Normalize Vector/1, Cross Product/2, [Rbc]
  Cross Product/1 -> Normalize Vector1/1
  [Rdc] -> Normalize Vector2/1, Cross Product/1
  Vector Concatenate/1 -> NQBb/1
  Normalize Vector/1 -> Vector Concatenate/1
  Normalize Vector2/1 -> Vector Concatenate/3
  Normalize Vector1/1 -> Vector Concatenate/2
  Demux1/1 -> Terminator5/1
  Demux3/1 -> Subtract2/3, Subtract1/3
  Demux3/2 -> Terminator7/1

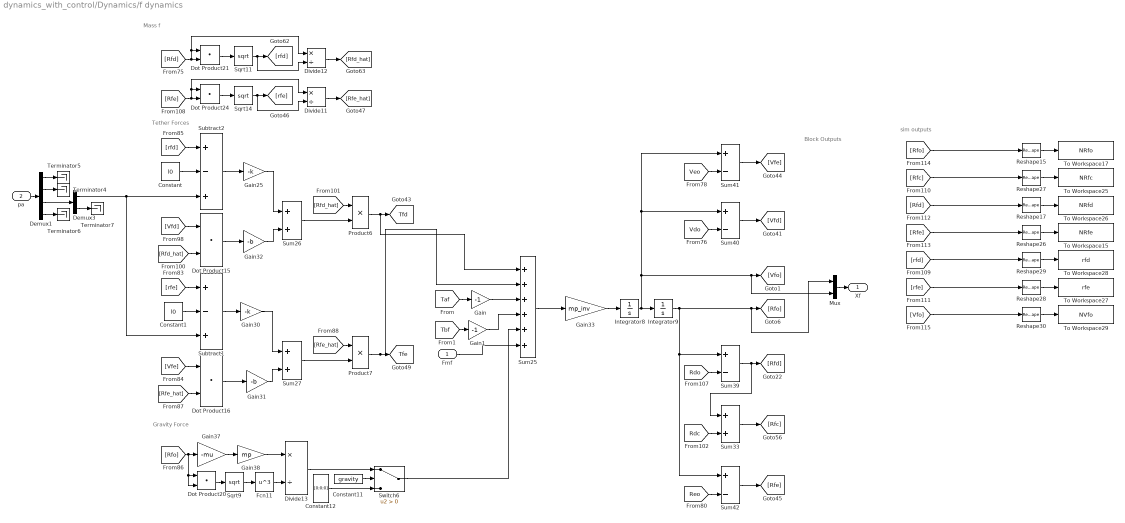
== system dynamics_with_control/Dynamics/f dynamics ==
  note: Block Outputs
  note: Mass f
  note: Tether Forces
  note: Gravity Force
  note: sim outputs
  Fmf : Inport
  pa : Inport  Port=2
  Constant : Constant  Value=l0
  Constant1 : Constant  Value=l0
  Constant11 : Constant  Value=gravity
  Constant12 : Constant  Value=[0;0;0]  VectorParams1D=off
  Demux1 : Demux
  Demux3 : Demux  Outputs=2
  Divide11 : Product  Inputs=*/
  Divide12 : Product  Inputs=*/
  Divide13 : Product  Inputs=*/
  Dot Product{15..16,20..21,24} (5 alike) : DotProduct  OutDataTypeStr=Inherit: Inherit via internal rule
  Fcn11 : Fcn  Expr=u^3
  Gain : Gain  Gain=-1
  Gain1 : Gain  Gain=-1
  Gain25 : Gain  Gain=-k
  Gain30 : Gain  Gain=-k
  Gain31 : Gain  Gain=-b
  Gain32 : Gain  Gain=-b
  Gain33 : Gain  Gain=mp_inv
  Gain37 : Gain  Gain=-mu
  Gain38 : Gain  Gain=mp
  Integrator8 : Integrator  InitialCondition=NVfo0
  Integrator9 : Integrator  InitialCondition=NRfo0
  Mux : Mux  Inputs=2
  Product6 : Product
  Product7 : Product
  Reshape{15,17,26..30} (7 alike) : Reshape
  Sqrt11 : Sqrt
  Sqrt14 : Sqrt
  Sqrt9 : Sqrt
  Subtract1 : Sum  Inputs=+-+
  Subtract2 : Sum  Inputs=+-+
  Sum25 : Sum  Inputs=++++++
  Sum26 : Sum
  Sum27 : Sum
  Sum33 : Sum
  Sum{39..42} (4 alike) : Sum  Inputs=+-
  Switch6 : Switch  Criteria=u2 > Threshold  SaturateOnIntegerOverflow=off  InputSameDT=off
  Terminator{4..7} (4 alike) : Terminator
  To Workspace15 : ToWorkspace  VariableName=NRfe  SampleTime=-1
  To Workspace17 : ToWorkspace  VariableName=NRfo  SampleTime=-1
      settings: Save2DSignal=2-D array (concatenate along first dimension)
  To Workspace25 : ToWorkspace  VariableName=NRfc  SampleTime=-1
      settings: Save2DSignal=2-D array (concatenate along first dimension)
  To Workspace26 : ToWorkspace  VariableName=NRfd  SampleTime=-1
  To Workspace27 : ToWorkspace  VariableName=rfe  SampleTime=-1
      settings: Save2DSignal=2-D array (concatenate along first dimension)
  To Workspace28 : ToWorkspace  VariableName=rfd  SampleTime=-1
      settings: Save2DSignal=2-D array (concatenate along first dimension)
  To Workspace29 : ToWorkspace  VariableName=NVfo  SampleTime=-1
      settings: Save2DSignal=2-D array (concatenate along first dimension)
  Xf : Outport
  tag scope: Tfd=global, Tfe=global
  wires:
  [Rdc] -> Sum33/2
  Sum27/1 -> Product7/2
  Divide12/1 -> [Rfd_hat]
  Divide13/1 -> Switch6/1
  Sum33/1 -> [Rfc]
  [Reo] -> Sum42/2
  Gain33/1 -> Integrator8/1
  Gain25/1 -> Sum26/1
  Sqrt11/1 -> Divide12/2, [rfd]
  Sum41/1 -> [Vfe]
  Switch6/1 -> Sum25/5
  Dot Product15/1 -> Gain32/1
  [Vfd] -> Dot Product15/1
  Dot Product21/1 -> Sqrt11/1
  Dot Product20/1 -> Sqrt9/1
  Constant12/1 -> Switch6/3
  [Rfd_hat] -> Dot Product15/2
  Dot Product24/1 -> Sqrt14/1
  [Vdo] -> Sum40/2
  [Veo] -> Sum41/2
  Gain31/1 -> Sum27/2
  [Rfo] -> Dot Product20/2, Dot Product20/1, Gain37/1
  [Rfd_hat] -> Product6/1
  [Rfe] -> Divide11/1, Dot Product24/1, Dot Product24/2
  Integrator9/1 -> Sum42/1, Sum39/1, Mux/1, [Rfo]
  Integrator8/1 -> Integrator9/1, Mux/2, [Vfo], Sum41/1, Sum40/1
  Sqrt9/1 -> Fcn11/1
  Product6/1 -> Sum25/1, [Tfd]
  Gain32/1 -> Sum26/2
  Product7/1 -> Sum25/2, [Tfe]
  [Rfe_hat] -> Dot Product16/2
  Sum40/1 -> [Vfd]
  Sum42/1 -> [Rfe]
  [Rdo] -> Sum39/2
  [Rfd] -> Divide12/1, Dot Product21/1, Dot Product21/2
  [Rfe_hat] -> Product7/1
  Gain37/1 -> Gain38/1
  Gain38/1 -> Divide13/1
  Sqrt14/1 -> Divide11/2, [rfe]
  Sum26/1 -> Product6/2
  Divide11/1 -> [Rfe_hat]
  Fcn11/1 -> Divide13/2
  Sum25/1 -> Gain33/1
  [Vfe] -> Dot Product16/1
  Sum39/1 -> Sum33/1, [Rfd]
  Gain30/1 -> Sum27/1
  Constant11/1 -> Switch6/2
  Dot Product16/1 -> Gain31/1
  Reshape26/1 -> To Workspace15/1
  [Vfo] -> Reshape30/1
  Reshape30/1 -> To Workspace29/1
  [Rfe] -> Reshape26/1
  Reshape27/1 -> To Workspace25/1
  [Rfd] -> Reshape17/1
  Reshape29/1 -> To Workspace28/1
  [rfe] -> Reshape28/1
  Reshape28/1 -> To Workspace27/1
  [Rfc] -> Reshape27/1
  [Rfo] -> Reshape15/1
  Reshape17/1 -> To Workspace26/1
  [rfd] -> Reshape29/1
  Reshape15/1 -> To Workspace17/1
  [Taf] -> Gain/1
  [Tbf] -> Gain1/1
  Gain/1 -> Sum25/3
  Gain1/1 -> Sum25/4
  Mux/1 -> Xf/1
  Fmf/1 -> Sum25/6
  Subtract2/1 -> Gain25/1
  [rfd] -> Subtract2/1
  Constant/1 -> Subtract2/2
  [rfe] -> Subtract1/1
  Constant1/1 -> Subtract1/2
  Subtract1/1 -> Gain30/1
  Demux1/4 -> Terminator6/1
  Demux1/1 -> Terminator5/1
  pa/1 -> Demux1/1
  Demux3/2 -> Terminator7/1
  Demux1/3 -> Demux3/1
  Demux1/2 -> Terminator4/1
  Demux3/1 -> Subtract1/3, Subtract2/3

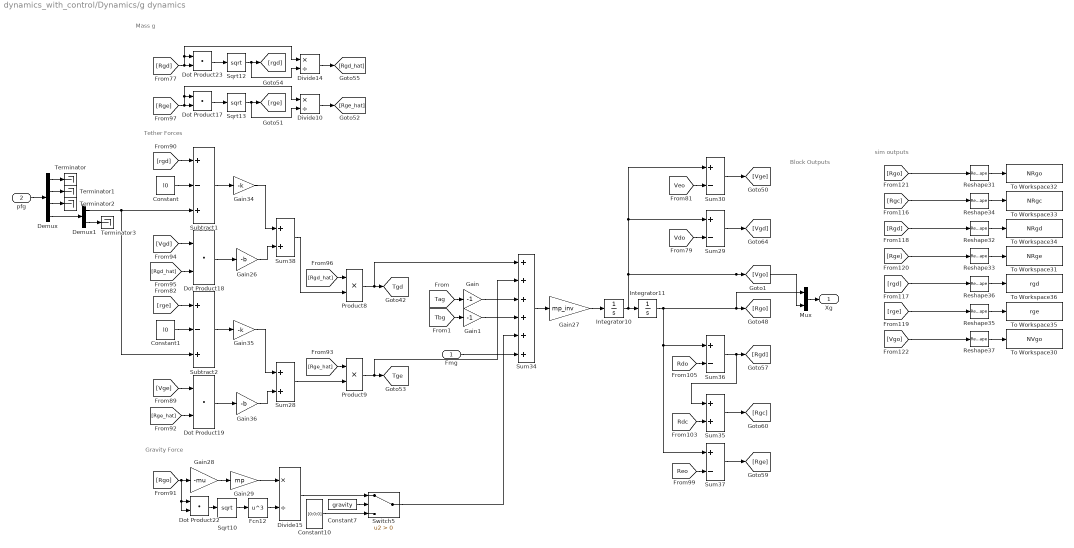
== system dynamics_with_control/Dynamics/g dynamics ==
  note: Block Outputs
  note: Mass g
  note: Tether Forces
  note: Gravity Force
  note: sim outputs
  Fmg : Inport
  pfg : Inport  Port=2
  Constant : Constant  Value=l0
  Constant1 : Constant  Value=l0
  Constant10 : Constant  Value=[0;0;0]  VectorParams1D=off
  Constant7 : Constant  Value=gravity
  Demux : Demux
  Demux1 : Demux  Outputs=2
  Divide10 : Product  Inputs=*/
  Divide14 : Product  Inputs=*/
  Divide15 : Product  Inputs=*/
  Dot Product{17..19,22..23} (5 alike) : DotProduct  OutDataTypeStr=Inherit: Inherit via internal rule
  Fcn12 : Fcn  Expr=u^3
  Gain : Gain  Gain=-1
  Gain1 : Gain  Gain=-1
  Gain26 : Gain  Gain=-b
  Gain27 : Gain  Gain=mp_inv
  Gain28 : Gain  Gain=-mu
  Gain29 : Gain  Gain=mp
  Gain34 : Gain  Gain=-k
  Gain35 : Gain  Gain=-k
  Gain36 : Gain  Gain=-b
  Integrator10 : Integrator  InitialCondition=NVgo0
  Integrator11 : Integrator  InitialCondition=NRgo0
  Mux : Mux  Inputs=2
  Product8 : Product
  Product9 : Product
  Reshape{31..37} (7 alike) : Reshape
  Sqrt10 : Sqrt
  Sqrt12 : Sqrt
  Sqrt13 : Sqrt
  Subtract1 : Sum  Inputs=+-+
  Subtract2 : Sum  Inputs=+-+
  Sum28 : Sum
  Sum{29..30,36..37} (4 alike) : Sum  Inputs=+-
  Sum34 : Sum  Inputs=++++++
  Sum35 : Sum
  Sum38 : Sum
  Switch5 : Switch  Criteria=u2 > Threshold  SaturateOnIntegerOverflow=off  InputSameDT=off
  Terminator{,1..3} (4 alike) : Terminator
  To Workspace30 : ToWorkspace  VariableName=NVgo  SampleTime=-1
      settings: Save2DSignal=2-D array (concatenate along first dimension)
  To Workspace31 : ToWorkspace  VariableName=NRge  SampleTime=-1
  To Workspace32 : ToWorkspace  VariableName=NRgo  SampleTime=-1
      settings: Save2DSignal=2-D array (concatenate along first dimension)
  To Workspace33 : ToWorkspace  VariableName=NRgc  SampleTime=-1
      settings: Save2DSignal=2-D array (concatenate along first dimension)
  To Workspace34 : ToWorkspace  VariableName=NRgd  SampleTime=-1
  To Workspace35 : ToWorkspace  VariableName=rge  SampleTime=-1
      settings: Save2DSignal=2-D array (concatenate along first dimension)
  To Workspace36 : ToWorkspace  VariableName=rgd  SampleTime=-1
      settings: Save2DSignal=2-D array (concatenate along first dimension)
  Xg : Outport
  tag scope: Tgd=global, Tge=global
  wires:
  Sum36/1 -> Sum35/1, [Rgd]
  Gain29/1 -> Divide15/1
  [Rge_hat] -> Product9/1
  Sum34/1 -> Gain27/1
  Sqrt10/1 -> Fcn12/1
  Dot Product22/1 -> Sqrt10/1
  [Veo] -> Sum30/2
  Switch5/1 -> Sum34/5
  Gain27/1 -> Integrator10/1
  Gain35/1 -> Sum28/1
  Fcn12/1 -> Divide15/2
  Product8/1 -> Sum34/1, [Tgd]
  [Vgd] -> Dot Product18/1
  Constant10/1 -> Switch5/3
  Gain34/1 -> Sum38/1
  Gain26/1 -> Sum38/2
  Product9/1 -> Sum34/2, [Tge]
  Sqrt13/1 -> Divide10/2, [rge]
  [Rge_hat] -> Dot Product19/2
  [Rgd_hat] -> Product8/1
  [Rgd] -> Divide14/1, Dot Product23/1, Dot Product23/2
  Divide15/1 -> Switch5/1
  Sum37/1 -> [Rge]
  [Rge] -> Divide10/1, Dot Product17/1, Dot Product17/2
  Sum38/1 -> Product8/2
  Integrator11/1 -> Sum36/1, Sum37/1, Mux/1, [Rgo]
  Sum28/1 -> Product9/2
  [Rdc] -> Sum35/2
  Constant7/1 -> Switch5/2
  Sum29/1 -> [Vgd]
  [Rgo] -> Dot Product22/2, Dot Product22/1, Gain28/1
  Gain28/1 -> Gain29/1
  Gain36/1 -> Sum28/2
  [Rgd_hat] -> Dot Product18/2
  [Rdo] -> Sum36/2
  Divide10/1 -> [Rge_hat]
  Sum30/1 -> [Vge]
  [Vge] -> Dot Product19/1
  [Reo] -> Sum37/2
  Divide14/1 -> [Rgd_hat]
  Dot Product23/1 -> Sqrt12/1
  Dot Product19/1 -> Gain36/1
  [Vdo] -> Sum29/2
  Dot Product18/1 -> Gain26/1
  Sum35/1 -> [Rgc]
  Sqrt12/1 -> Divide14/2, [rgd]
  Dot Product17/1 -> Sqrt13/1
  Reshape33/1 -> To Workspace31/1
  Reshape37/1 -> To Workspace30/1
  Reshape36/1 -> To Workspace36/1
  Reshape31/1 -> To Workspace32/1
  [Rgc] -> Reshape34/1
  [rge] -> Reshape35/1
  [rgd] -> Reshape36/1
  [Rgo] -> Reshape31/1
  [Rgd] -> Reshape32/1
  Reshape32/1 -> To Workspace34/1
  Reshape35/1 -> To Workspace35/1
  Reshape34/1 -> To Workspace33/1
  [Rge] -> Reshape33/1
  [Vgo] -> Reshape37/1
  Integrator10/1 -> Integrator11/1, Sum30/1, Sum29/1, Mux/2, [Vgo]
  [Tag] -> Gain/1
  Gain/1 -> Sum34/3
  [Tbg] -> Gain1/1
  Gain1/1 -> Sum34/4
  Mux/1 -> Xg/1
  Fmg/1 -> Sum34/6
  [rgd] -> Subtract1/1
  pfg/1 -> Demux/1
  Demux/2 -> Terminator1/1
  Demux/1 -> Terminator/1
  Constant/1 -> Subtract1/2
  Subtract1/1 -> Gain34/1
  [rge] -> Subtract2/1
  Constant1/1 -> Subtract2/2
  Subtract2/1 -> Gain35/1
  Demux/3 -> Terminator2/1
  Demux/4 -> Demux1/1
  Demux1/1 -> Subtract1/3, Subtract2/3
  Demux1/2 -> Terminator3/1

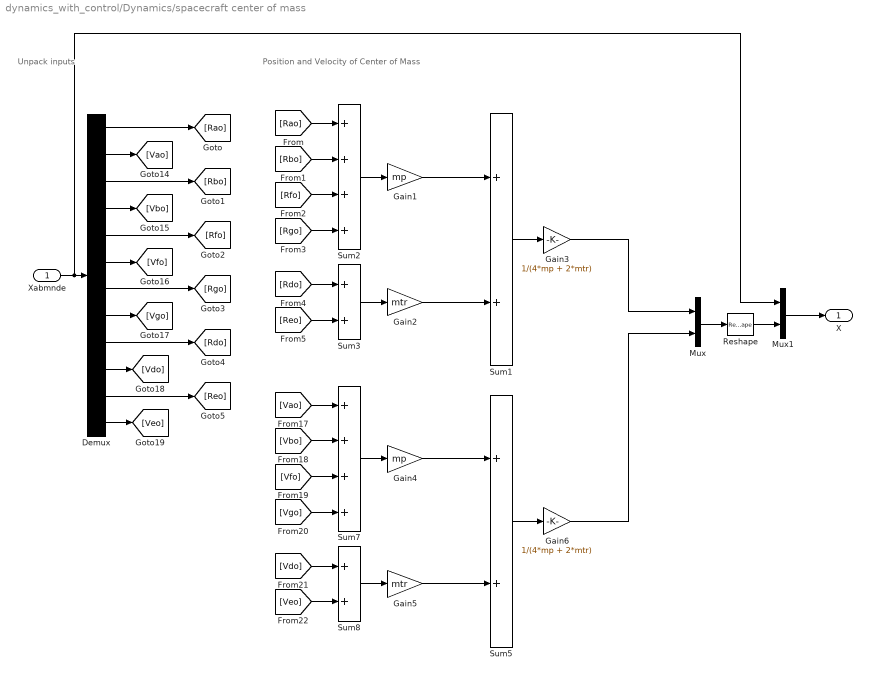
== system dynamics_with_control/Dynamics/spacecraft center of mass ==
  note: Position and Velocity of Center of Mass
  note: Unpack inputs
  Xabmnde : Inport
  Demux : Demux  Outputs=12
  Gain1 : Gain  Gain=mp
  Gain2 : Gain  Gain=mtr
  Gain3 : Gain  Gain=1/(4*mp + 2*mtr)
  Gain4 : Gain  Gain=mp
  Gain5 : Gain  Gain=mtr
  Gain6 : Gain  Gain=1/(4*mp + 2*mtr)
  Mux : Mux  Inputs=2
  Mux1 : Mux  Inputs=2
  Reshape : Reshape  OutputDimensionality=Customize  OutputDimensions=[6,1]
  Sum{1,3,5,8} (4 alike) : Sum
  Sum2 : Sum  Inputs=++++
  Sum7 : Sum  Inputs=++++
  X : Outport
  wires:
  [Vdo] -> Sum8/1
  [Vbo] -> Sum7/2
  Sum7/1 -> Gain4/1
  Gain2/1 -> Sum1/2
  [Vgo] -> Sum7/4
  [Rdo] -> Sum3/1
  Gain5/1 -> Sum5/2
  [Rfo] -> Sum2/3
  [Rbo] -> Sum2/2
  Sum8/1 -> Gain5/1
  Gain4/1 -> Sum5/1
  Sum5/1 -> Gain6/1
  [Vfo] -> Sum7/3
  [Rgo] -> Sum2/4
  Sum3/1 -> Gain2/1
  Sum1/1 -> Gain3/1
  Sum2/1 -> Gain1/1
  [Veo] -> Sum8/2
  [Reo] -> Sum3/2
  [Vao] -> Sum7/1
  [Rao] -> Sum2/1
  Gain1/1 -> Sum1/1
  Demux/12 -> [Veo]
  Xabmnde/1 -> Mux1/1, Demux/1
  Demux/5 -> [Rfo]
  Demux/3 -> [Rbo]
  Demux/6 -> [Vfo]
  Demux/10 -> [Vdo]
  Demux/8 -> [Vgo]
  Demux/9 -> [Rdo]
  Demux/7 -> [Rgo]
  Demux/2 -> [Vao]
  Demux/1 -> [Rao]
  Demux/11 -> [Reo]
  Demux/4 -> [Vbo]
  Gain3/1 -> Mux/1
  Gain6/1 -> Mux/2
  Mux/1 -> Reshape/1
  Mux1/1 -> X/1
  Reshape/1 -> Mux1/2

== system dynamics_with_control/Tether Length Controller/PD A ==
  lref : Inport
  a : Inport  Port=2
  Clock1 : Clock
  Clock2 : Clock
  Constant : Constant  Value=0
  Demux : Demux  Outputs=2
  Integrator2 : Integrator  Commented=on
  Sum1 : Sum  Inputs=|+-
  Sum2 : Sum  Inputs=+++
  Sum3 : Sum  Inputs=|+-
  Switch1 : Switch  Criteria=u2 > Threshold  Threshold=StopTime/2  SaturateOnIntegerOverflow=off  InputSameDT=off
  Switch2 : Switch  Criteria=u2 > Threshold  Threshold=StopTime/2  SaturateOnIntegerOverflow=off  InputSameDT=off
  kd : Gain  Gain=-.01
  ki : Gain  Commented=on  Gain=.01
  kp : Gain  Gain=-1e-3
  u : Outport
  wires:
  Integrator2/1 -> ki/1
  kd/1 -> Sum2/3
  kp/1 -> Sum2/1
  ki/1 -> Sum2/2
  Sum2/1 -> u/1
  Sum1/1 -> kp/1, Integrator2/1
  Switch1/1 -> Sum1/1
  lref/1 -> Switch1/1
  Clock1/1 -> Switch1/2
  a/1 -> Demux/1
  Demux/1 -> Switch1/3, Sum1/2
  Demux/2 -> Switch2/3, Sum3/2
  Constant/1 -> Switch2/1
  Clock2/1 -> Switch2/2
  Switch2/1 -> Sum3/1
  Sum3/1 -> kd/1

== system dynamics_with_control/Tether Length Controller/PD B ==
  lref : Inport
  b : Inport  Port=2
  Clock1 : Clock
  Clock2 : Clock
  Constant1 : Constant  Value=0
  Demux : Demux  Outputs=2
  Integrator2 : Integrator  Commented=on
  Sum1 : Sum  Inputs=|+-
  Sum2 : Sum  Inputs=+++
  Sum3 : Sum  Inputs=|+-
  Switch1 : Switch  Criteria=u2 > Threshold  Threshold=StopTime/2  SaturateOnIntegerOverflow=off  InputSameDT=off
  Switch2 : Switch  Criteria=u2 > Threshold  Threshold=StopTime/2  SaturateOnIntegerOverflow=off  InputSameDT=off
  kd : Gain  Gain=-0.01
  ki : Gain  Commented=on  Gain=.01
  kp : Gain  Gain=-1e-3
  u : Outport
  wires:
  Integrator2/1 -> ki/1
  kd/1 -> Sum2/3
  kp/1 -> Sum2/1
  ki/1 -> Sum2/2
  Sum2/1 -> u/1
  Sum1/1 -> kp/1, Integrator2/1
  Switch1/1 -> Sum1/1
  lref/1 -> Switch1/1
  Clock1/1 -> Switch1/2
  b/1 -> Demux/1
  Demux/1 -> Switch1/3, Sum1/2
  Clock2/1 -> Switch2/2
  Demux/2 -> Switch2/3, Sum3/2
  Constant1/1 -> Switch2/1
  Switch2/1 -> Sum3/1
  Sum3/1 -> kd/1

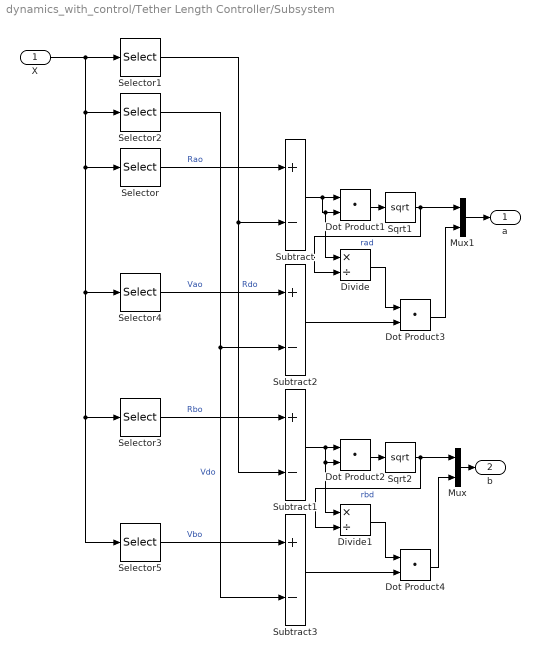
== system dynamics_with_control/Tether Length Controller/Subsystem ==
  X : Inport
  Divide : Product  Inputs=*/
  Divide1 : Product  Inputs=*/
  Dot Product{1..4} (4 alike) : DotProduct  OutDataTypeStr=Inherit: Inherit via internal rule
  Mux : Mux  Inputs=2
  Mux1 : Mux  Inputs=2
  Selector : Selector  NumberOfDimensions=2  InputPortWidth=3  IndexOptions=Index vector (dialog),Index vector (dialog)  Indices=[1 2 3],1  OutputSizes=1,1
  Selector1 : Selector  NumberOfDimensions=2  InputPortWidth=3  IndexOptions=Index vector (dialog),Index vector (dialog)  Indices=[25 26 27],1  OutputSizes=1,1
  Selector2 : Selector  NumberOfDimensions=2  InputPortWidth=3  IndexOptions=Index vector (dialog),Index vector (dialog)  Indices=[28 29 30],1  OutputSizes=1,1
  Selector3 : Selector  NumberOfDimensions=2  InputPortWidth=3  IndexOptions=Index vector (dialog),Index vector (dialog)  Indices=[7 8 9],1  OutputSizes=1,1
  Selector4 : Selector  NumberOfDimensions=2  InputPortWidth=3  IndexOptions=Index vector (dialog),Index vector (dialog)  Indices=[4 5 6],1  OutputSizes=1,1
  Selector5 : Selector  NumberOfDimensions=2  InputPortWidth=3  IndexOptions=Index vector (dialog),Index vector (dialog)  Indices=[10 11 12],1  OutputSizes=1,1
  Sqrt1 : Sqrt
  Sqrt2 : Sqrt
  Subtract{,1..3} (4 alike) : Sum  Inputs=+-
  a : Outport
  b : Outport  Port=2
  wires:
  Selector/1 -> Subtract/1  "Rao"
  Selector5/1 -> Subtract3/1  "Vbo"
  Selector3/1 -> Subtract1/1  "Rbo"
  Selector1/1 -> Subtract1/2, Subtract/2  "Rdo"
  Mux1/1 -> a/1
  Sqrt2/1 -> Divide1/2, Mux/1  "rbd"
  X/1 -> Selector5/1, Selector3/1, Selector4/1, Selector/1, Selector2/1, Selector1/1
  Selector4/1 -> Subtract2/1  "Vao"
  Subtract1/1 -> Divide1/1, Dot Product2/2, Dot Product2/1
  Dot Product2/1 -> Sqrt2/1
  Subtract/1 -> Divide/1, Dot Product1/2, Dot Product1/1
  Dot Product1/1 -> Sqrt1/1
  Selector2/1 -> Subtract2/2, Subtract3/2  "Vdo"
  Sqrt1/1 -> Divide/2, Mux1/1  "rad"
  Mux/1 -> b/1
  Subtract2/1 -> Dot Product3/2
  Divide/1 -> Dot Product3/1
  Dot Product3/1 -> Mux1/2
  Divide1/1 -> Dot Product4/1
  Subtract3/1 -> Dot Product4/2
  Dot Product4/1 -> Mux/2

== matlab function dynamics_with_control/Anguar Momentum Controller/get magnetic field ==
  data: r input; B output
function B = fcn(r)
    mu0 = 1.25663706212e-6; % N*A^-2
    mE = -8e22*[0;0;1]; % A*m^2
    B = (mu0/(4*pi))*(((3*r*dot(mE,r))./norm(r)^5 - mE./norm(r)^3));
end

== matlab function dynamics_with_control/Anguar Momentum Controller/Skew Symmetric ==
  data: u input; y output
function y = fcn(u)

y = [0    -u(3)  u(2);
     u(3)  0    -u(1);
    -u(2)  u(1)  0   ];

== matlab function dynamics_with_control/Anguar Momentum Controller/Skew Symmetric1 ==
  data: u input; y output
function y = fcn(u)

y = [0    -u(3)  u(2);
     u(3)  0    -u(1);
    -u(2)  u(1)  0   ];

== matlab function dynamics_with_control/Anguar Momentum Controller/Skew Symmetric2 ==
  data: u input; y output
function y = fcn(u)

y = [0    -u(3)  u(2);
     u(3)  0    -u(1);
    -u(2)  u(1)  0   ];

== matlab function dynamics_with_control/Anguar Momentum Controller/Skew Symmetric3 ==
  data: u input; y output
function y = fcn(u)

y = [0    -u(3)  u(2);
     u(3)  0    -u(1);
    -u(2)  u(1)  0   ];

== matlab function dynamics_with_control/Anguar Momentum Controller/blkdiag ==
  data: A input; y output; B input; C input; D input
function y = fcn(A, B, C, D)

y = blkdiag(A, B, C, D);

== matlab function dynamics_with_control/Anguar Momentum Controller/pinv ==
  data: u input; y output
function y = fcn(u)

y = pinv(u);

== matlab function dynamics_with_control/Dynamics/MATLAB Function ==
  data: BQO input; q output; qprev input
function q = dcm2quat(BQO, qprev)
switch max([abs(BQO(1,1)),abs(BQO(2,2)),abs(BQO(3,3)),abs(trace(BQO))])
    case abs(BQO(1,1))
        q1 = 1 + 2*BQO(1,1) - trace(BQO);
        q2 = BQO(1,2) + BQO(2,1);
        q3 = BQO(1,3) + BQO(3,1);
        q4 = BQO(2,3) - BQO(3,2);
    case abs(BQO(2,2))
        q1 = BQO(2,1) + BQO(1,2);
        q2 = 1 + 2*BQO(2,2) - trace(BQO);
        q3 = BQO(2,3) + BQO(3,2);
        q4 = BQO(3,1) - BQO(1,3);
    case abs(BQO(3,3))
        q1 = BQO(3,1) + BQO(1,3);
        q2 = BQO(3,2) + BQO(2,3);
        q3 = 1 + 2*BQO(3,3) - trace(BQO);
        q4 = BQO(1,2) - BQO(2,1);
    otherwise
        q1 = BQO(2,3) - BQO(3,2);
        q2 = BQO(3,1) - BQO(1,3);
        q3 = BQO(1,2) - BQO(2,1);
        q4 = 1 + trace(BQO);
end
q = [q1;q2;q3;q4]./norm([q1;q2;q3;q4]);
if dot(q,qprev) < 0
    q = q*-1;
end

== matlab function dynamics_with_control/Dynamics/MATLAB Function1 ==
  data: BQO input; q output; qprev input
function q = dcm2quat(BQO, qprev)
switch max([abs(BQO(1,1)),abs(BQO(2,2)),abs(BQO(3,3)),abs(trace(BQO))])
    case abs(BQO(1,1))
        q1 = 1 + 2*BQO(1,1) - trace(BQO);
        q2 = BQO(1,2) + BQO(2,1);
        q3 = BQO(1,3) + BQO(3,1);
        q4 = BQO(2,3) - BQO(3,2);
    case abs(BQO(2,2))
        q1 = BQO(2,1) + BQO(1,2);
        q2 = 1 + 2*BQO(2,2) - trace(BQO);
        q3 = BQO(2,3) + BQO(3,2);
        q4 = BQO(3,1) - BQO(1,3);
    case abs(BQO(3,3))
        q1 = BQO(3,1) + BQO(1,3);
        q2 = BQO(3,2) + BQO(2,3);
        q3 = 1 + 2*BQO(3,3) - trace(BQO);
        q4 = BQO(1,2) - BQO(2,1);
    otherwise
        q1 = BQO(2,3) - BQO(3,2);
        q2 = BQO(3,1) - BQO(1,3);
        q3 = BQO(1,2) - BQO(2,1);
        q4 = 1 + trace(BQO);
end
q = [q1;q2;q3;q4]./norm([q1;q2;q3;q4]);
if dot(q,qprev) < 0
    q = q*-1;
end
